simulink model "NEXTCAR_Interface"  (R2017a)
settings: Solver=ode4  StartTime=0.0  StopTime=10000  FixedStep=0.001  RelTol=1e-3  EnableMultiTasking=on
undefined symbols (not defined in the file or in its folder): IO306
libraries: NEXTCAR_Library x50, speedgoatlib_IO106 x4, slrtlib x3, simulink x3, speedgoatlib_fpga_pwm x2, speedgoatlib_IO204 x2, slrttcplib x2, simulink_extras x2, speedgoatlib_fpga x1, xpcseriallib x1, powerlib_meascontrol x1
(part 2 of 2)

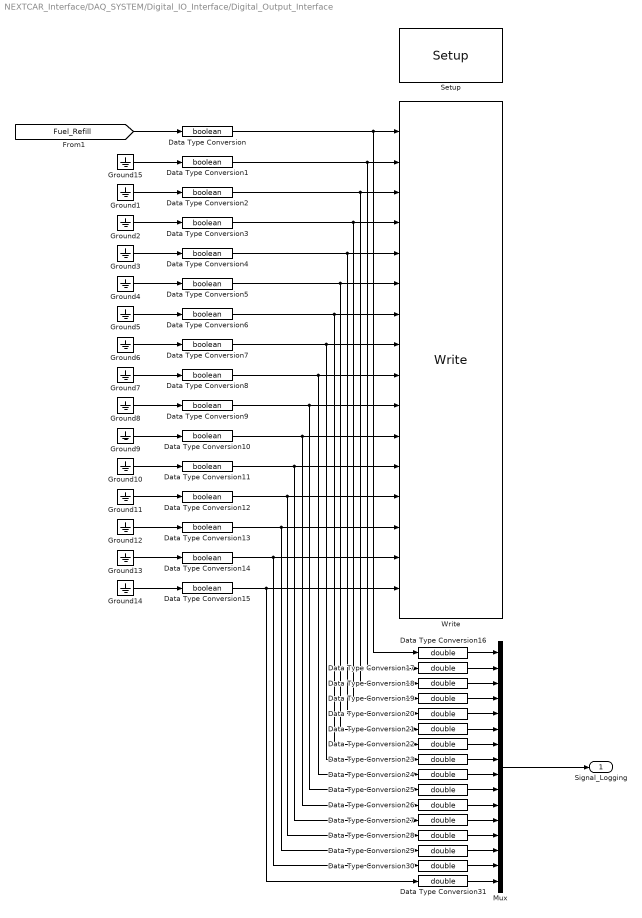
== system NEXTCAR_Interface/DAQ_SYSTEM/Digital_IO_Interface/Digital_Output_Interface ==
  Data Type Conversion{,1..15} (16 alike) : DataTypeConversion  OutDataTypeStr=boolean
  Data Type Conversion{16..31} (16 alike) : DataTypeConversion  OutDataTypeStr=double
  Ground{1..15} (15 alike) : Ground
  Mux : Mux  Inputs=16
  Setup : speedgoatlib_IO204/Setup  group=Module setup  id=1  pciSlot=-1  debounceEnable=off  debounceValue=0.001  reset=[0]  value=[0]
      settings: SourceProductName=Simulink Real-Time: Speedgoat I/O Driver Library
  Write : speedgoatlib_IO204/Write  id=1  portType=16 ports of type boolean  ts=-1  pciSlot=-1
      settings: SourceProductName=Simulink Real-Time: Speedgoat I/O Driver Library
  Signal_Logging : Outport
  wires:
  Ground9/1 -> Data Type Conversion10/1
  Ground12/1 -> Data Type Conversion13/1
  Ground13/1 -> Data Type Conversion14/1
  Ground4/1 -> Data Type Conversion5/1
  Ground7/1 -> Data Type Conversion8/1
  Ground14/1 -> Data Type Conversion15/1
  Ground11/1 -> Data Type Conversion12/1
  [Fuel_Refill] -> Data Type Conversion/1
  Ground10/1 -> Data Type Conversion11/1
  Ground15/1 -> Data Type Conversion1/1
  Ground8/1 -> Data Type Conversion9/1
  Ground2/1 -> Data Type Conversion3/1
  Ground3/1 -> Data Type Conversion4/1
  Ground5/1 -> Data Type Conversion6/1
  Data Type Conversion16/1 -> Mux/1
  Data Type Conversion18/1 -> Mux/3
  Data Type Conversion25/1 -> Mux/10
  Data Type Conversion27/1 -> Mux/12
  Data Type Conversion28/1 -> Mux/13
  Data Type Conversion2/1 -> Data Type Conversion18/1, Write/3
  Data Type Conversion9/1 -> Data Type Conversion25/1, Write/10
  Data Type Conversion17/1 -> Mux/2
  Ground6/1 -> Data Type Conversion7/1
  Data Type Conversion8/1 -> Data Type Conversion24/1, Write/9
  Data Type Conversion5/1 -> Data Type Conversion21/1, Write/6
  Data Type Conversion12/1 -> Data Type Conversion28/1, Write/13
  Data Type Conversion14/1 -> Data Type Conversion30/1, Write/15
  Data Type Conversion15/1 -> Data Type Conversion31/1, Write/16
  Data Type Conversion6/1 -> Data Type Conversion22/1, Write/7
  Data Type Conversion3/1 -> Data Type Conversion19/1, Write/4
  Ground1/1 -> Data Type Conversion2/1
  Data Type Conversion10/1 -> Data Type Conversion26/1, Write/11
  Mux/1 -> Signal_Logging/1
  Data Type Conversion19/1 -> Mux/4
  Data Type Conversion11/1 -> Data Type Conversion27/1, Write/12
  Data Type Conversion13/1 -> Data Type Conversion29/1, Write/14
  Data Type Conversion20/1 -> Mux/5
  Data Type Conversion21/1 -> Mux/6
  Data Type Conversion22/1 -> Mux/7
  Data Type Conversion4/1 -> Data Type Conversion20/1, Write/5
  Data Type Conversion1/1 -> Data Type Conversion17/1, Write/2
  Data Type Conversion23/1 -> Mux/8
  Data Type Conversion24/1 -> Mux/9
  Data Type Conversion/1 -> Data Type Conversion16/1, Write/1
  Data Type Conversion7/1 -> Data Type Conversion23/1, Write/8
  Data Type Conversion26/1 -> Mux/11
  Data Type Conversion29/1 -> Mux/14
  Data Type Conversion31/1 -> Mux/16
  Data Type Conversion30/1 -> Mux/15

== system NEXTCAR_Interface/DAQ_SYSTEM/Logging_Interface/CPL_Data_Logging ==
  Logging_Data : Inport
  Enable : EnablePort  StatesWhenEnabling=reset
  "Scope " : slrtlib/Displays and Logging/Scope   scopeno=3  scopetype=File  autostart=on  viewmode=Graphical redraw  formatstr='%15.6f'  grid=on  ylimits=[0,0]  nosamples=200000  noprepostsamples=0  interleave=1  triggermode=FreeRun  triggersignal=1  trigsignalfromport=on  triggerlevel=0.5  triggerslope=Rising  triggerscope=1  triggersample=0  filename=CplLog.dat  mode=Commit  writesize=512  autorestart=off  dynamicfilemode=off  maxwritefilesize=512*1024^2
  wires:
  Logging_Data/1 -> "Scope "/1

== system NEXTCAR_Interface/DAQ_SYSTEM/Logging_Interface/Timer ==
  incr_condition : Inport
  target_time : Inport  Port=2
  reset : Inport  Port=3
  Constant : Constant  Value=0
  Constant1 : Constant  Value=0
  Constant2 : Constant
  MinMax : MinMax  Inputs=2
  Relational Operator : RelationalOperator  Operator=<  OutDataTypeStr=boolean  RndMeth=Simplest
  Subtract : Sum
  Subtract1 : Sum  Inputs=-+
  Switch1 : Switch  Criteria=u2 > Threshold
  Switch2 : Switch  Criteria=u2 > Threshold
  Unit Delay : UnitDelay  SampleTime=-1
  timer_status : Outport
  wires:
  Switch1/1 -> Subtract/2
  Constant/1 -> Switch1/3
  incr_condition/1 -> Switch1/2
  Constant2/1 -> Relational Operator/2, Switch1/1
  Constant1/1 -> Switch2/1
  Switch2/1 -> Subtract1/1, Unit Delay/1
  Unit Delay/1 -> Subtract/1
  reset/1 -> Switch2/2
  MinMax/1 -> Switch2/3
  Subtract/1 -> MinMax/1
  target_time/1 -> Subtract1/2, MinMax/2
  Subtract1/1 -> Relational Operator/1
  Relational Operator/1 -> timer_status/1

== system NEXTCAR_Interface/DAQ_SYSTEM/Logging_Interface/Trigger2 ==
  System_Clock : Inport
  Constant : Constant
  Divide : Product  Inputs=*/
  Floor : Rounding
  Memory : Memory  InheritSampleTime=on
  Relational Operator : RelationalOperator  Operator=>  OutDataTypeStr=boolean  RndMeth=Simplest
  Trigger : Outport
  wires:
  System_Clock/1 -> Divide/1
  Relational Operator/1 -> Trigger/1
  Divide/1 -> Floor/1
  Memory/1 -> Relational Operator/2
  Constant/1 -> Divide/2
  Floor/1 -> Memory/1, Relational Operator/1

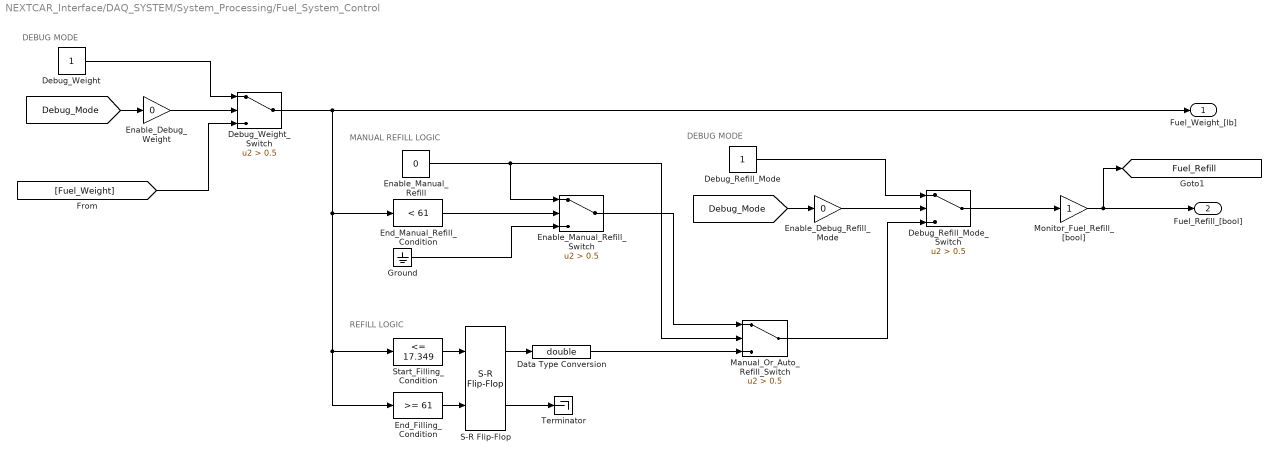
== system NEXTCAR_Interface/DAQ_SYSTEM/System_Processing/Fuel_System_Control ==
  note: REFILL LOGIC
  note: MANUAL REFILL LOGIC
  note: DEBUG MODE
  note: DEBUG MODE
  Data Type Conversion : DataTypeConversion  OutDataTypeStr=double
  Debug_Refill_Mode : Constant
  Debug_Refill_Mode_Switch : Switch  Criteria=u2 > Threshold  Threshold=0.5
  Debug_Weight : Constant
  Debug_Weight_Switch : Switch  Criteria=u2 > Threshold  Threshold=0.5
  Enable_Debug_Refill_Mode : Gain  Gain=0
  Enable_Debug_Weight : Gain  Gain=0
  Enable_Manual_Refill : Constant  Value=0  OutDataTypeStr=boolean
  Enable_Manual_Refill_Switch : Switch  Criteria=u2 > Threshold  Threshold=0.5
  End_Filling_Condition : simulink/Logic and Bit Operations/Compare To Constant  relop=>=  const=61  OutDataTypeStr=boolean
  End_Manual_Refill_Condition : simulink/Logic and Bit Operations/Compare To Constant  relop=<  const=61  OutDataTypeStr=boolean
  Ground : Ground
  Manual_Or_Auto_Refill_Switch : Switch  Criteria=u2 > Threshold  Threshold=0.5
  Monitor_Fuel_Refill_[bool] : Gain
  S-R Flip-Flop : simulink_extras/Flip Flops/S-R Flip-Flop  initial_condition=0
  Start_Filling_Condition : simulink/Logic and Bit Operations/Compare To Constant  relop=<=  const=17.349  OutDataTypeStr=boolean
  Terminator : Terminator
  Fuel_Weight_[lb] : Outport
  Fuel_Refill_[bool] : Outport  Port=2
  tag scope: Fuel_Refill=global
  wires:
  Data Type Conversion/1 -> Manual_Or_Auto_Refill_Switch/3
  Enable_Manual_Refill_Switch/1 -> Manual_Or_Auto_Refill_Switch/1
  Debug_Weight_Switch/1 -> Fuel_Weight_[lb]/1, Start_Filling_Condition/1, End_Filling_Condition/1, End_Manual_Refill_Condition/1
  End_Filling_Condition/1 -> S-R Flip-Flop/2
  Enable_Debug_Refill_Mode/1 -> Debug_Refill_Mode_Switch/2
  S-R Flip-Flop/2 -> Terminator/1
  Start_Filling_Condition/1 -> S-R Flip-Flop/1
  [Debug_Mode] -> Enable_Debug_Refill_Mode/1
  S-R Flip-Flop/1 -> Data Type Conversion/1
  Debug_Weight/1 -> Debug_Weight_Switch/1
  Ground/1 -> Enable_Manual_Refill_Switch/3
  Manual_Or_Auto_Refill_Switch/1 -> Debug_Refill_Mode_Switch/3
  Enable_Debug_Weight/1 -> Debug_Weight_Switch/2
  End_Manual_Refill_Condition/1 -> Enable_Manual_Refill_Switch/2
  Debug_Refill_Mode_Switch/1 -> Monitor_Fuel_Refill_[bool]/1
  [Debug_Mode] -> Enable_Debug_Weight/1
  Enable_Manual_Refill/1 -> Enable_Manual_Refill_Switch/1, Manual_Or_Auto_Refill_Switch/2
  [Fuel_Weight] -> Debug_Weight_Switch/3
  Debug_Refill_Mode/1 -> Debug_Refill_Mode_Switch/1
  Monitor_Fuel_Refill_[bool]/1 -> Fuel_Refill_[bool]/1, [Fuel_Refill]

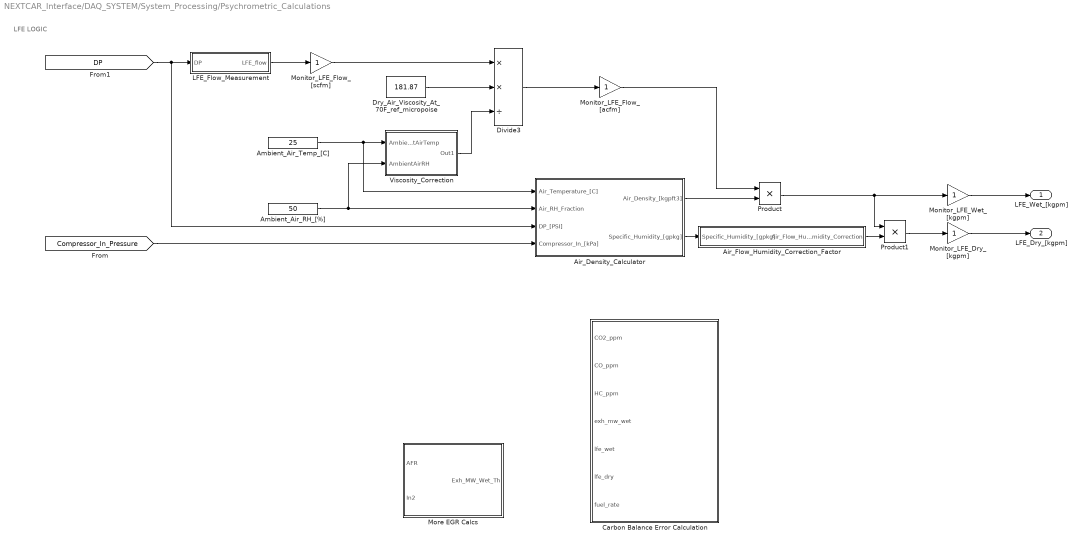
== system NEXTCAR_Interface/DAQ_SYSTEM/System_Processing/Psychrometric_Calculations ==
  note: LFE LOGIC
  Air_Density_Calculator : Subsystem
  Air_Flow_Humidity_Correction_Factor : Subsystem
  Ambient_Air_RH_[%] : Constant  Value=50
  Ambient_Air_Temp_[C] : Constant  Value=25
  Carbon Balance Error Calculation : Subsystem
  Divide3 : Product  Inputs=**/
  Dry_Air_Viscosity_At_70F_ref_micropoise : Constant  Value=181.87
  LFE_Flow_Measurement : Subsystem
  Monitor_LFE_Dry_[kgpm] : Gain
  Monitor_LFE_Flow_[acfm] : Gain
  Monitor_LFE_Flow_[scfm] : Gain
  Monitor_LFE_Wet_[kgpm] : Gain
  More EGR Calcs : Subsystem
  Product : Product  RndMeth=Zero
  Product1 : Product  RndMeth=Zero
  Viscosity_Correction : Subsystem
  LFE_Wet_[kgpm] : Outport
  LFE_Dry_[kgpm] : Outport  Port=2
  wires:
  Product/1 -> Monitor_LFE_Wet_[kgpm]/1, Product1/1
  Monitor_LFE_Flow_[scfm]/1 -> Divide3/1
  Ambient_Air_RH_[%]/1 -> Air_Density_Calculator/2(Air_RH_Fraction), Viscosity_Correction/2(AmbientAirRH)
  Ambient_Air_Temp_[C]/1 -> Viscosity_Correction/1(AmbientAirTemp), Air_Density_Calculator/1(Air_Temperature_[C])
  Monitor_LFE_Wet_[kgpm]/1 -> LFE_Wet_[kgpm]/1
  Divide3/1 -> Monitor_LFE_Flow_[acfm]/1
  Dry_Air_Viscosity_At_70F_ref_micropoise/1 -> Divide3/2
  Viscosity_Correction/1(Out1) -> Divide3/3
  [DP] -> LFE_Flow_Measurement/1(DP), Air_Density_Calculator/3(DP_[PSI])
  [Compressor_In_Pressure] -> Air_Density_Calculator/4(Compressor_In_[kPa])
  Monitor_LFE_Flow_[acfm]/1 -> Product/1
  Air_Density_Calculator/1(Air_Density_[kgpft3]) -> Product/2
  LFE_Flow_Measurement/1(LFE_flow) -> Monitor_LFE_Flow_[scfm]/1
  Air_Density_Calculator/2(Specific_Humidity_[gpkg]) -> Air_Flow_Humidity_Correction_Factor/1(Specific_Humidity_[gpkg])
  Air_Flow_Humidity_Correction_Factor/1(Air_Flow_Humidity_Correction) -> Product1/2
  Product1/1 -> Monitor_LFE_Dry_[kgpm]/1
  Monitor_LFE_Dry_[kgpm]/1 -> LFE_Dry_[kgpm]/1

== system NEXTCAR_Interface/DAQ_SYSTEM/Analog_IO_Interface/Fuel_Measurements/Fuel_Weight ==
  note: FUEL WEIGHT CONVERSION
  Voltage : Inport
  "FuelBucketOffset  " : Constant  Value=16.16
  "OffsetVoltage " : Constant  Value=1.8826
  "ProportionalVoltage " : Gain  Gain=10.009
  Sum : Sum  Inputs=|+-
  Sum1 : Sum  Inputs=|+-
  Weight : Outport
  wires:
  Voltage/1 -> "ProportionalVoltage "/1
  "OffsetVoltage "/1 -> Sum/2
  "ProportionalVoltage "/1 -> Sum/1
  Sum/1 -> Sum1/1
  Sum1/1 -> Weight/1
  "FuelBucketOffset  "/1 -> Sum1/2

== system NEXTCAR_Interface/DAQ_SYSTEM/Analog_IO_Interface/LFE_Measurements/LFE_Linear_Sensor_Calibration ==
  In1 : Inport
  Calibration Constant 1 : Gain  Gain=slope  SaturateOnIntegerOverflow=on  OutDataTypeStr=Inherit: Same as input  ParamDataTypeStr=Inherit: Same as input
  Calibration Constant 2 : Constant  Value=offset
  Sum1 : Sum  Inputs=|++  SaturateOnIntegerOverflow=on  InputSameDT=on  OutDataTypeStr=Inherit: Same as first input
  Out1 : Outport
  wires:
  Calibration Constant 2/1 -> Sum1/2
  Calibration Constant 1/1 -> Sum1/1
  In1/1 -> Calibration Constant 1/1
  Sum1/1 -> Out1/1

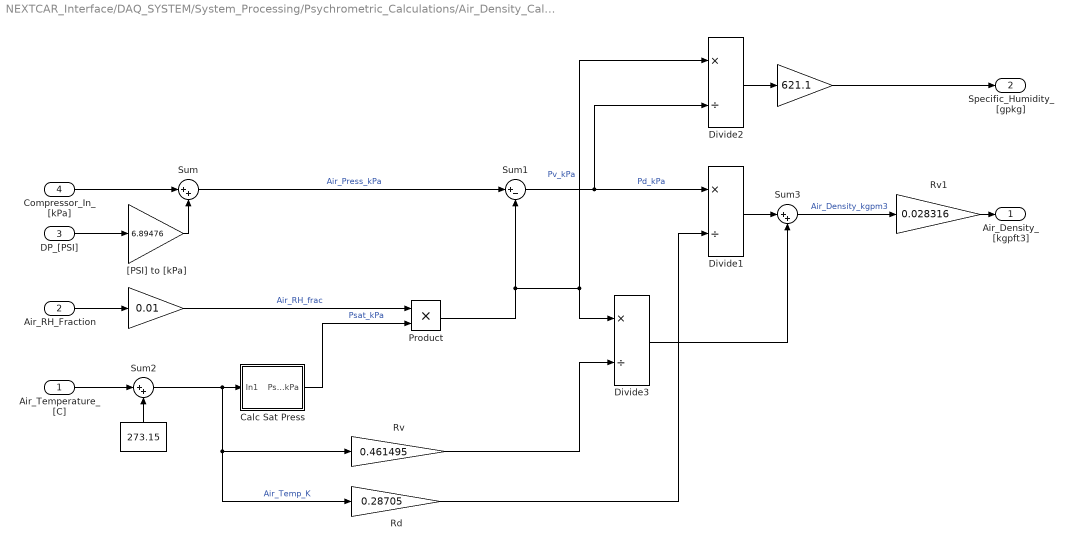
== system NEXTCAR_Interface/DAQ_SYSTEM/System_Processing/Psychrometric_Calculations/Air_Density_Calculator ==
  Air_Temperature_[C] : Inport
  Air_RH_Fraction : Inport  Port=2
  DP_[PSI] : Inport  Port=3
  Compressor_In_[kPa] : Inport  Port=4
  " " : Constant  Value=273.15
  "     " : Gain  Gain=0.01
  "        " : Gain  Gain=621.1
  Calc Sat Press : Subsystem
  Divide1 : Product  Inputs=*/
  Divide2 : Product  Inputs=*/
  Divide3 : Product  Inputs=*/
  Product : Product  RndMeth=Zero
  Rd : Gain  Gain=0.28705
  Rv : Gain  Gain=0.461495
  Rv1 : Gain  Gain=0.028316
  Sum : Sum  Inputs=|++
  Sum1 : Sum  Inputs=|+-
  Sum2 : Sum  Inputs=|++
  Sum3 : Sum  Inputs=|++
  "[PSI] to [kPa]" : Gain  Gain=6.89476
  Air_Density_[kgpft3] : Outport
  Specific_Humidity_[gpkg] : Outport  Port=2
  wires:
  Air_RH_Fraction/1 -> "     "/1
  "     "/1 -> Product/1  "Air_RH_frac"
  Sum2/1 -> Calc Sat Press/1(In1), Rv/1, Rd/1  "Air_Temp_K"
  Air_Temperature_[C]/1 -> Sum2/1
  " "/1 -> Sum2/2
  Calc Sat Press/1(Psat_kPa) -> Product/2  "Psat_kPa"
  Product/1 -> Sum1/2, Divide3/1, Divide2/1  "Pv_kPa"
  Sum1/1 -> Divide1/1, Divide2/2  "Pd_kPa"
  Rv/1 -> Divide3/2
  Rd/1 -> Divide1/2
  Divide3/1 -> Sum3/2
  Divide1/1 -> Sum3/1
  Sum3/1 -> Rv1/1  "Air_Density_kgpm3"
  Rv1/1 -> Air_Density_[kgpft3]/1
  Divide2/1 -> "        "/1
  "        "/1 -> Specific_Humidity_[gpkg]/1
  Compressor_In_[kPa]/1 -> Sum/1
  "[PSI] to [kPa]"/1 -> Sum/2
  DP_[PSI]/1 -> "[PSI] to [kPa]"/1
  Sum/1 -> Sum1/1  "Air_Press_kPa"

== system NEXTCAR_Interface/DAQ_SYSTEM/System_Processing/Psychrometric_Calculations/Air_Flow_Humidity_Correction_Factor ==
  Specific_Humidity_[gpkg] : Inport
  Air_Press_mbar : Constant  Value=1000
  Divide2 : Product  Inputs=*/
  Sum2 : Sum  Inputs=++|
  Air_Flow_Humidity_Correction : Outport
  wires:
  Specific_Humidity_[gpkg]/1 -> Sum2/2
  Sum2/1 -> Divide2/2
  Air_Press_mbar/1 -> Divide2/1, Sum2/1
  Divide2/1 -> Air_Flow_Humidity_Correction/1

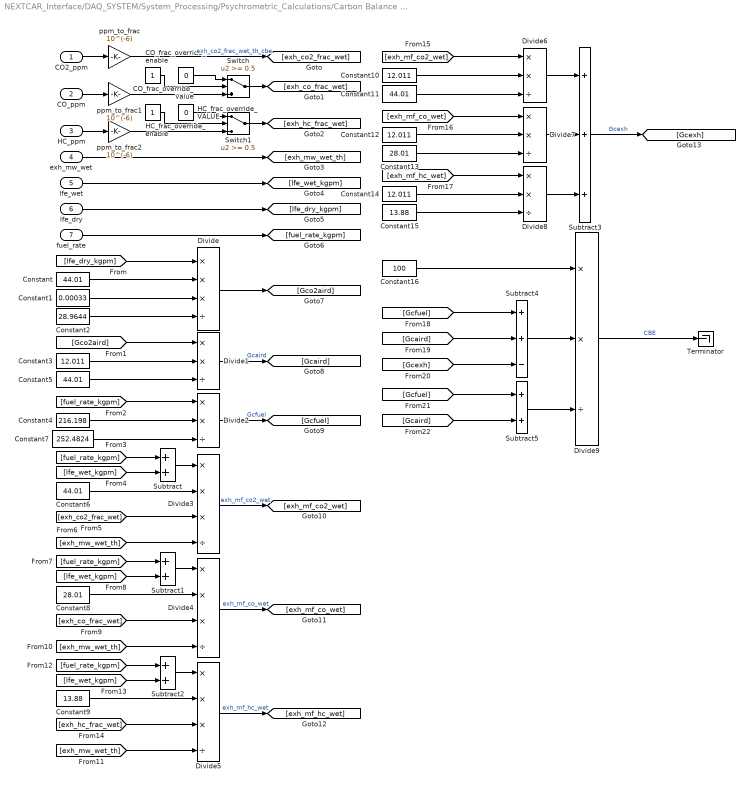
== system NEXTCAR_Interface/DAQ_SYSTEM/System_Processing/Psychrometric_Calculations/Carbon Balance Error Calculation ==
  CO2_ppm : Inport
  CO_ppm : Inport  Port=2
  HC_ppm : Inport  Port=3
  exh_mw_wet : Inport  Port=4
  lfe_wet : Inport  Port=5
  lfe_dry : Inport  Port=6
  fuel_rate : Inport  Port=7
  CO_frac_override_enable : Constant
  CO_frac_override_value : Constant  Value=0
  Constant{,5..6,11} (4 alike) : Constant  Value=44.01
  Constant1 : Constant  Value=0.00033
  Constant{3,10,12,14} (4 alike) : Constant  Value=12.011
  Constant13 : Constant  Value=28.01
  Constant15 : Constant  Value=13.88
  Constant16 : Constant  Value=100
  Constant2 : Constant  Value=28.9644
  Constant4 : Constant  Value=216.198
  Constant7 : Constant  Value=252.4824
  Constant8 : Constant  Value=28.01
  Constant9 : Constant  Value=13.88
  Divide{,3..5} (4 alike) : Product  Inputs=***/
  Divide{1..2,6..9} (6 alike) : Product  Inputs=**/
  HC_frac_override_VALUE : Constant  Value=0
  HC_frac_override_enable : Constant
  Subtract{,1..2,5} (4 alike) : Sum
  Subtract3 : Sum  Inputs=+++
  Subtract4 : Sum  Inputs=++-
  Switch : Switch  Threshold=0.5
  Switch1 : Switch  Threshold=0.5
  Terminator : Terminator
  ppm_to_frac : Gain  Gain=10^(-6)
  ppm_to_frac1 : Gain  Gain=10^(-6)
  ppm_to_frac2 : Gain  Gain=10^(-6)
  wires:
  CO2_ppm/1 -> ppm_to_frac/1
  ppm_to_frac/1 -> [exh_co2_frac_wet]  "exh_co2_frac_wet_th_cbe"
  CO_ppm/1 -> ppm_to_frac1/1
  HC_ppm/1 -> ppm_to_frac2/1
  ppm_to_frac1/1 -> Switch/3
  Switch/1 -> [exh_co_frac_wet]
  CO_frac_override_enable/1 -> Switch/2
  CO_frac_override_value/1 -> Switch/1
  ppm_to_frac2/1 -> Switch1/3
  HC_frac_override_enable/1 -> Switch1/2
  HC_frac_override_VALUE/1 -> Switch1/1
  Switch1/1 -> [exh_hc_frac_wet]
  exh_mw_wet/1 -> [exh_mw_wet_th]
  lfe_wet/1 -> [lfe_wet_kgpm]
  lfe_dry/1 -> [lfe_dry_kgpm]
  fuel_rate/1 -> [fuel_rate_kgpm]
  [lfe_dry_kgpm] -> Divide/1
  Constant/1 -> Divide/2
  Constant1/1 -> Divide/3
  Constant2/1 -> Divide/4
  Divide/1 -> [Gco2aird]
  [Gco2aird] -> Divide1/1
  Constant3/1 -> Divide1/2
  Divide1/1 -> [Gcaird]  "Gcaird"
  Constant5/1 -> Divide1/3
  [fuel_rate_kgpm] -> Divide2/1
  Constant4/1 -> Divide2/2
  Divide2/1 -> [Gcfuel]  "Gcfuel"
  Constant7/1 -> Divide2/3
  [fuel_rate_kgpm] -> Subtract/1
  [lfe_wet_kgpm] -> Subtract/2
  Subtract/1 -> Divide3/1
  Constant6/1 -> Divide3/2
  [exh_co2_frac_wet] -> Divide3/3
  [exh_mw_wet_th] -> Divide3/4
  Divide3/1 -> [exh_mf_co2_wet]  "exh_mf_co2_wet"
  [fuel_rate_kgpm] -> Subtract1/1
  [lfe_wet_kgpm] -> Subtract1/2
  Subtract1/1 -> Divide4/1
  Constant8/1 -> Divide4/2
  [exh_co_frac_wet] -> Divide4/3
  [exh_mw_wet_th] -> Divide4/4
  Divide4/1 -> [exh_mf_co_wet]  "exh_mf_co_wet"
  [fuel_rate_kgpm] -> Subtract2/1
  [lfe_wet_kgpm] -> Subtract2/2
  Subtract2/1 -> Divide5/1
  Constant9/1 -> Divide5/2
  [exh_hc_frac_wet] -> Divide5/3
  [exh_mw_wet_th] -> Divide5/4
  Divide5/1 -> [exh_mf_hc_wet]  "exh_mf_hc_wet"
  [exh_mf_co2_wet] -> Divide6/1
  Constant10/1 -> Divide6/2
  Constant11/1 -> Divide6/3
  [exh_mf_co_wet] -> Divide7/1
  Constant12/1 -> Divide7/2
  Constant13/1 -> Divide7/3
  [exh_mf_hc_wet] -> Divide8/1
  Constant14/1 -> Divide8/2
  Constant15/1 -> Divide8/3
  Divide6/1 -> Subtract3/1
  Divide7/1 -> Subtract3/2
  Divide8/1 -> Subtract3/3
  Subtract3/1 -> [Gcexh]  "Gcexh"
  [Gcfuel] -> Subtract4/1
  [Gcaird] -> Subtract4/2
  [Gcexh] -> Subtract4/3
  [Gcfuel] -> Subtract5/1
  [Gcaird] -> Subtract5/2
  Constant16/1 -> Divide9/1
  Subtract4/1 -> Divide9/2
  Subtract5/1 -> Divide9/3
  Divide9/1 -> Terminator/1  "CBE"

== system NEXTCAR_Interface/DAQ_SYSTEM/System_Processing/Psychrometric_Calculations/LFE_Flow_Measurement ==
  DP : Inport
  Gain : Gain  Gain=27.6799
  Quadratic Sensor Calibration1 : Subsystem  mask{cubic_coef=5.8882783e-2, quad_coef=-1.9680047, lin_coef=1.3406752e2, offset=0}
      mask prompts: cubic_coef "Cubic Coefficient?"; quad_coef "Quadratic coefficient?"; lin_coef "Linear Coefficient?"; offset "Offset (in units)?"
      mask init:
      | str1 = ['[A]x^3 = ' num2str(cubic_coef)];
      | str2 = ['[B]x^2 = ' num2str(quad_coef)];
      | str3 = ['[C]x = ' num2str(lin_coef)];
      | str4 = ['[D] = ' num2str(offset)];
      mask Display:
      | text(0.5, 0.2, str4, 'horizontalAlignment', 'center','verticalAlignment', 'middle')
      | text(0.5, 0.4, str3, 'horizontalAlignment', 'center', 'verticalAlignment', 'middle')
      | text(0.5, 0.6, str2, 'horizontalAlignment', 'center', 'verticalAlignment', 'middle')
      | text(0.5, 0.8, str1, 'horizontalAlignment', 'center', 'verticalAlignment', 'middle')
  LFE_flow : Outport
  wires:
  Quadratic Sensor Calibration1/1(Out1) -> LFE_flow/1  "LFE_flow"
  Gain/1 -> Quadratic Sensor Calibration1/1(In1)  "LFE_delta_P_inH2O"
  DP/1 -> Gain/1

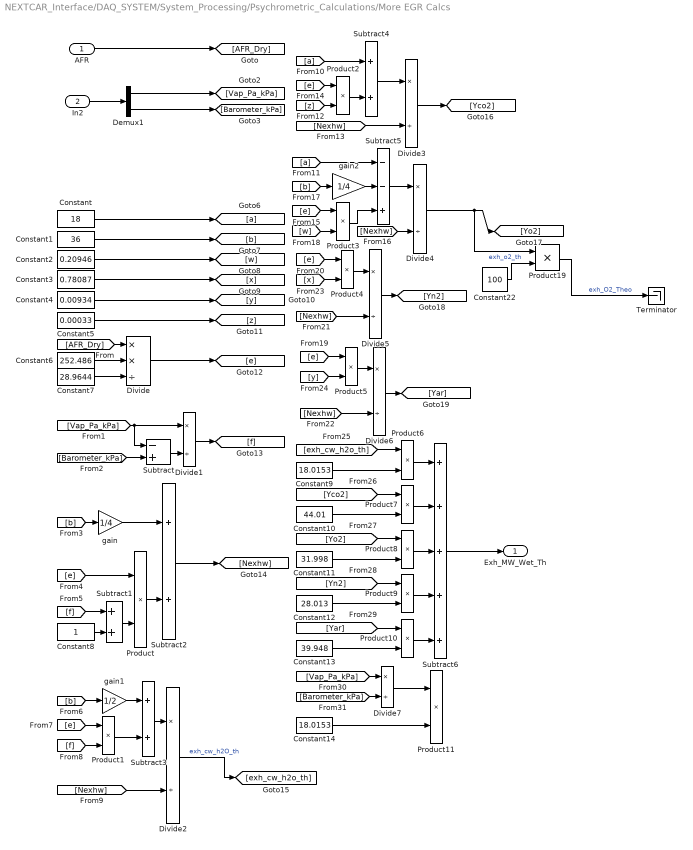
== system NEXTCAR_Interface/DAQ_SYSTEM/System_Processing/Psychrometric_Calculations/More EGR Calcs ==
  AFR : Inport
  In2 : Inport  Port=2
  Constant : Constant  Value=18
  Constant1 : Constant  Value=36
  Constant10 : Constant  Value=44.01
  Constant11 : Constant  Value=31.998
  Constant12 : Constant  Value=28.013
  Constant13 : Constant  Value=39.948
  Constant14 : Constant  Value=18.0153
  Constant2 : Constant  Value=0.20946
  Constant22 : Constant  Value=100
  Constant3 : Constant  Value=0.78087
  Constant4 : Constant  Value=0.00934
  Constant5 : Constant  Value=0.00033
  Constant6 : Constant  Value=252.486
  Constant7 : Constant  Value=28.9644
  Constant8 : Constant
  Constant9 : Constant  Value=18.0153
  Demux1 : Demux  Outputs=2
  Divide : Product  Inputs=**/
  Divide{1..7} (7 alike) : Product  Inputs=*/
  Product{,1..11,19} (13 alike) : Product  RndMeth=Zero
  Subtract : Sum  Inputs=-+
  Subtract{1..4} (4 alike) : Sum
  Subtract5 : Sum  Inputs=--+
  Subtract6 : Sum  Inputs=+++++
  Terminator : Terminator
  gain : Gain  Gain=1/4
  gain1 : Gain  Gain=1/2
  gain2 : Gain  Gain=1/4
  Exh_MW_Wet_Th : Outport
  wires:
  AFR/1 -> [AFR_Dry]
  In2/1 -> Demux1/1
  Demux1/1 -> [Vap_Pa_kPa]
  Demux1/2 -> [Barometer_kPa]
  Constant/1 -> [a]
  Constant1/1 -> [b]
  Constant2/1 -> [w]
  Constant3/1 -> [x]
  Constant4/1 -> [y]
  Constant5/1 -> [z]
  Constant7/1 -> Divide/3
  Constant6/1 -> Divide/2
  [AFR_Dry] -> Divide/1
  Divide/1 -> [e]
  [Vap_Pa_kPa] -> Divide1/1, Subtract/1
  Subtract/1 -> Divide1/2
  [Barometer_kPa] -> Subtract/2
  Divide1/1 -> [f]
  [b] -> gain/1
  [f] -> Subtract1/1
  Constant8/1 -> Subtract1/2
  [e] -> Product/1
  Subtract1/1 -> Product/2
  gain/1 -> Subtract2/1
  Product/1 -> Subtract2/2
  Subtract2/1 -> [Nexhw]
  [b] -> gain1/1
  [e] -> Product1/1
  [f] -> Product1/2
  gain1/1 -> Subtract3/1
  Product1/1 -> Subtract3/2
  Subtract3/1 -> Divide2/1
  [Nexhw] -> Divide2/2
  Divide2/1 -> [exh_cw_h2o_th]  "exh_cw_h2O_th"
  [e] -> Product2/1
  [z] -> Product2/2
  [a] -> Subtract4/1
  Product2/1 -> Subtract4/2
  Subtract4/1 -> Divide3/1
  [Nexhw] -> Divide3/2
  Divide3/1 -> [Yco2]
  [a] -> Subtract5/1
  gain2/1 -> Subtract5/2
  [Nexhw] -> Divide4/2
  [b] -> gain2/1
  Divide4/1 -> [Yo2], Product19/1  "exh_o2_th"
  [e] -> Product3/1
  [w] -> Product3/2
  Product3/1 -> Subtract5/3
  Subtract5/1 -> Divide4/1
  [Nexhw] -> Divide5/2
  Divide5/1 -> [Yn2]
  [e] -> Product4/1
  [x] -> Product4/2
  Product4/1 -> Divide5/1
  [Nexhw] -> Divide6/2
  Divide6/1 -> [Yar]
  [e] -> Product5/1
  [y] -> Product5/2
  Product5/1 -> Divide6/1
  [exh_cw_h2o_th] -> Product6/1
  Constant9/1 -> Product6/2
  [Yco2] -> Product7/1
  Constant10/1 -> Product7/2
  [Yo2] -> Product8/1
  Constant11/1 -> Product8/2
  [Yn2] -> Product9/1
  Constant12/1 -> Product9/2
  [Yar] -> Product10/1
  Constant13/1 -> Product10/2
  Product6/1 -> Subtract6/1
  Product7/1 -> Subtract6/2
  Product8/1 -> Subtract6/3
  Product9/1 -> Subtract6/4
  Product10/1 -> Subtract6/5
  Subtract6/1 -> Exh_MW_Wet_Th/1
  [Vap_Pa_kPa] -> Divide7/1
  [Barometer_kPa] -> Divide7/2
  Divide7/1 -> Product11/1
  Constant14/1 -> Product11/2
  Constant22/1 -> Product19/2
  Product19/1 -> Terminator/1  "exh_O2_Theo"

== system NEXTCAR_Interface/DAQ_SYSTEM/System_Processing/Psychrometric_Calculations/Viscosity_Correction ==
  AmbientAirTemp : Inport
  AmbientAirRH : Inport  Port=2
  Constant1 : Constant  Value=273.15
  Constant2 : Constant  Value=3/2
  Constant3 : Constant  Value=14.58
  Constant4 : Constant  Value=110.4
  Divide4 : Product  Inputs=*/
  Lookup Table (2-D) : Lookup2D  RowIndex="[10.00\t15.56\t21.11\t26.67\t32.22\t37.78\t43.33\t48.89\t54.44\t60.00\t65.56]"  ColumnIndex="[10\t20\t30\t40\t50\t60\t70\t80\t90]"  Table="[1.0000\t1.0000\t1.0000\t1.0000\t1.0000\t1.0000\t1.0000\t1.0000\t1.0000;1.0000\t1.0000\t1.0000\t1.0000\t1.0000\t1.0000\t0.9990\t0.9989\t0.9988;1.0000\t1.0000\t1.0000\t1.0000\t0.9990\t0.9988\t0.9985\t0.9980\t0.9975;1.0000\t0.9996\t0.9993\t0.9989\t0.9985\t0.9980\t0.9975\t0.9963\t0.9950;0.9996\t0.9991\t0.9985\t0.9980\t0.9975\t0.9963\t0.9950\t0.9938\t0.9925;0.9993\t0.9986\t0.9980\t0.9970\t0.9960\t0.9943\t0.9925\t0.9913\t0.9900;0.9989\t0.9979\t0.9968\t0.9952\t0.9935\t0.9918\t0.9900\t0.9888\t0.9875;0.9986\t0.9973\t0.9960\t0.9938\t0.9915\t0.9895\t0.9875\t0.9850\t0.9825;0.9982\t0.9961\t0.9940\t0.9920\t0.9900\t0.9863\t0.9825\t0.9800\t0.9775;0.9979\t0.9952\t0.9925\t0.9888\t0.9850\t0.9813\t0.9775\t0.9725\t0.9675;0.9975\t0.9938\t0.9900\t0.9850\t0.9800\t0.9738\t0.9675\t0.9613\t0.9550]"  LookUpMeth=Interpolation-Use End Values
  Math Function : Math  Operator=pow  SaturateOnIntegerOverflow=on
  Product1 : Product  RndMeth=Zero
  Product2 : Product  RndMeth=Zero
  Subtract : Sum
  Subtract1 : Sum
  Out1 : Outport
  wires:
  AmbientAirTemp/1 -> Lookup Table (2-D)/1, Subtract/2
  Constant1/1 -> Subtract/1
  Subtract/1 -> [AAT_degK]
  [AAT_degK] -> Math Function/1
  Constant2/1 -> Math Function/2
  Math Function/1 -> Product1/1
  Constant3/1 -> Product1/2
  Product1/1 -> Divide4/1
  Subtract1/1 -> Divide4/2
  [AAT_degK] -> Subtract1/1
  Constant4/1 -> Subtract1/2
  Divide4/1 -> Product2/1
  Lookup Table (2-D)/1 -> Product2/2
  Product2/1 -> Out1/1
  AmbientAirRH/1 -> Lookup Table (2-D)/2

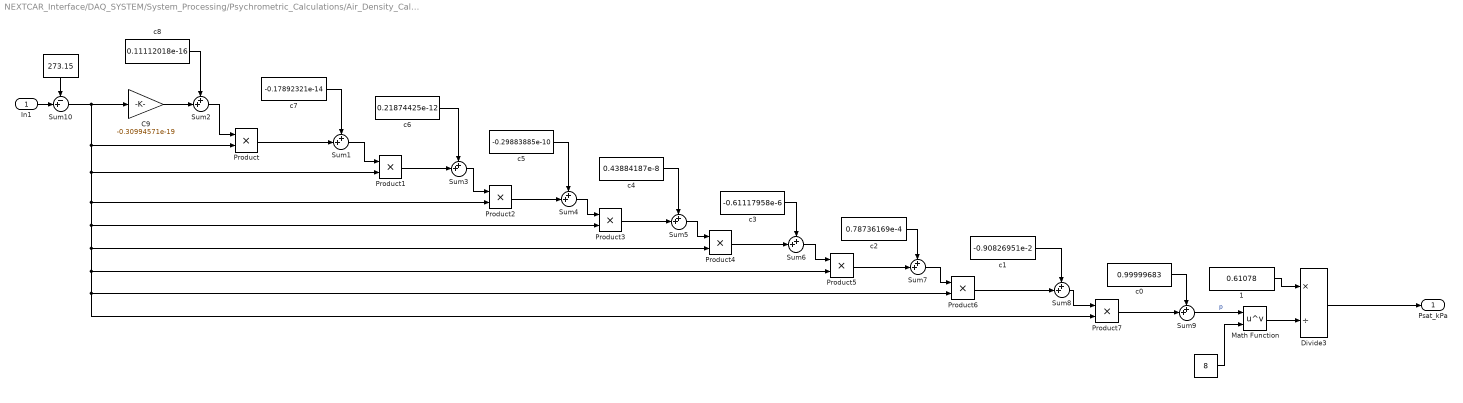
== system NEXTCAR_Interface/DAQ_SYSTEM/System_Processing/Psychrometric_Calculations/Air_Density_Calculator/Calc Sat Press ==
  In1 : Inport
  " " : Constant  Value=8
  "  " : Constant  Value=273.15
  " 1" : Constant  Value=0.61078
  C9 : Gain  Gain=-0.30994571e-19
  Divide3 : Product  Inputs=*/
  Math Function : Math  Operator=pow  SaturateOnIntegerOverflow=on
  Product{,1..7} (8 alike) : Product  RndMeth=Zero
  Sum{1..9} (9 alike) : Sum  Inputs=++|
  Sum10 : Sum  Inputs=-+|
  c0 : Constant  Value=0.99999683
  c1 : Constant  Value=-0.90826951e-2
  c2 : Constant  Value=0.78736169e-4
  c3 : Constant  Value=-0.61117958e-6
  c4 : Constant  Value=0.43884187e-8
  c5 : Constant  Value=-0.29883885e-10
  c6 : Constant  Value=0.21874425e-12
  c7 : Constant  Value=-0.17892321e-14
  c8 : Constant  Value=0.11112018e-16
  Psat_kPa : Outport
  wires:
  Divide3/1 -> Psat_kPa/1
  C9/1 -> Sum2/2
  c8/1 -> Sum2/1
  Sum2/1 -> Product/1
  Product/1 -> Sum1/2
  c7/1 -> Sum1/1
  Sum1/1 -> Product1/1
  Product1/1 -> Sum3/2
  c6/1 -> Sum3/1
  Sum3/1 -> Product2/1
  Product2/1 -> Sum4/2
  c5/1 -> Sum4/1
  Sum4/1 -> Product3/1
  Product3/1 -> Sum5/2
  c4/1 -> Sum5/1
  Sum5/1 -> Product4/1
  Product4/1 -> Sum6/2
  c3/1 -> Sum6/1
  Sum6/1 -> Product5/1
  Product5/1 -> Sum7/2
  c2/1 -> Sum7/1
  Sum7/1 -> Product6/1
  Product6/1 -> Sum8/2
  c1/1 -> Sum8/1
  Sum8/1 -> Product7/1
  Product7/1 -> Sum9/2
  c0/1 -> Sum9/1
  Math Function/1 -> Divide3/2
  " 1"/1 -> Divide3/1
  " "/1 -> Math Function/2
  Sum9/1 -> Math Function/1  "p"
  Sum10/1 -> C9/1, Product/2, Product1/2, Product2/2, Product3/2, Product4/2, Product5/2, Product6/2, Product7/2
  In1/1 -> Sum10/2
  "  "/1 -> Sum10/1

== system NEXTCAR_Interface/DAQ_SYSTEM/System_Processing/Psychrometric_Calculations/LFE_Flow_Measurement/Quadratic Sensor Calibration1 ==
  In1 : Inport
  Cubic Coefficient : Gain  Gain=cubic_coef  SaturateOnIntegerOverflow=on  OutDataTypeStr=Inherit: Same as input  ParamDataTypeStr=Inherit: Same as input
  Linear Coefficient : Gain  Gain=lin_coef  SaturateOnIntegerOverflow=on  OutDataTypeStr=Inherit: Same as input  ParamDataTypeStr=Inherit: Same as input
  Offset Constant : Constant  Value=offset
  Product : Product  SaturateOnIntegerOverflow=on  RndMeth=Zero  InputSameDT=on  OutDataTypeStr=Inherit: Same as first input
  Product1 : Product  Inputs=3  SaturateOnIntegerOverflow=on  RndMeth=Zero  InputSameDT=on  OutDataTypeStr=Inherit: Same as first input
  Quadratic Coefficient : Gain  Gain=quad_coef  SaturateOnIntegerOverflow=on  OutDataTypeStr=Inherit: Same as input  ParamDataTypeStr=Inherit: Same as input
  Sum1 : Sum  Inputs=++++  SaturateOnIntegerOverflow=on  InputSameDT=on  OutDataTypeStr=Inherit: Same as first input
  Out1 : Outport
  wires:
  Cubic Coefficient/1 -> Sum1/4
  Product1/1 -> Cubic Coefficient/1
  Product/1 -> Quadratic Coefficient/1
  Quadratic Coefficient/1 -> Sum1/1
  In1/1 -> Product/1, Product1/1, Product1/2, Product1/3, Product/2, Linear Coefficient/1
  Linear Coefficient/1 -> Sum1/2
  Offset Constant/1 -> Sum1/3
  Sum1/1 -> Out1/1
